simulink model "Lixivaition_model"  (R2025b)
settings: Solver=VariableStepAuto  StartTime=0.0  StopTime=200  RelTol=1e-3
values from neighbouring files (symbols this model uses):
  k = data.k_sharpness    [Hydrocyclone.m]    (also in closed_circuit_mill_cyclone.m; closed_circuit_with_pulp.m = 2.5)
undefined symbols (not defined in the file or in its folder): C0, Ceq
settings Model: Creator=fabri  LastModifiedBy=fabri

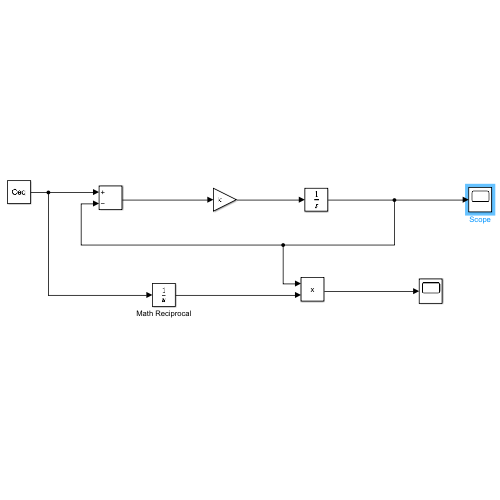
[thumbnail: Simulink's stored preview of the top-level diagram]
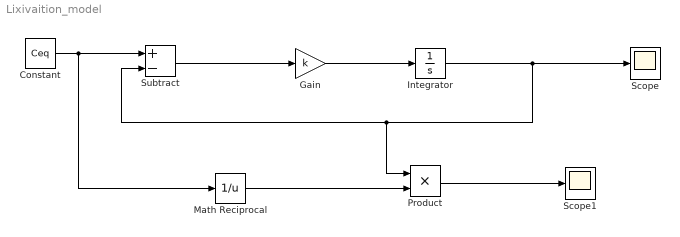
== system Lixivaition_model ==
  Constant : Constant  Value=Ceq
  Gain : Gain  Gain=k
  Integrator : Integrator  InitialCondition=C0
  Math Reciprocal : Math  Operator=reciprocal  SignedPower=on
  Product : Product
  Scope : Scope
      settings: ActiveDisplayYMinimum=-845.86969336603784  ActiveDisplayYMaximum=788.65250170399622
  Scope1 : Scope
      settings: ActiveDisplayYMinimum=-1.8430116415267102  ActiveDisplayYMaximum=1.7926392333478485
  Subtract : Sum  Inputs=+-
  wires:
  Integrator/1 -> Subtract/2, Product/1, Scope/1
  Gain/1 -> Integrator/1
  Subtract/1 -> Gain/1
  Constant/1 -> Math Reciprocal/1, Subtract/1
  Product/1 -> Scope1/1
  Math Reciprocal/1 -> Product/2
